simulink model "s_alqrd2"  (Simulink 4.00)
settings: Solver=ode45  SolverMode=SingleTasking  StartTime=0.0  StopTime=20  FixedStep=0.1  MaxStep=0.1  RelTol=1e-3  AbsTol=1e-6
values from neighbouring files (symbols this model uses):
  C = [Cp, zeros(1,ns)]    [akalm1.m]    (also in kalm1.m = my_sys1.c; kalm2.m = my_sys1.c; kalm3.m = my_sys1.c; kalm4.m = [eye(3,3), zeros(3,3)])
  F = K*(x_un/x_un(1))/kq1    [abeob1.m]    (also in akalm1.m = xp_un*alpha; alqr1.m = K*(x_un/x_un(1))/k1; alqrd1.m = K*(x_un/x_un(1))/k1; apol1.m = K*(x_un/x_un(1))/k1)
  k1 = K(1)    [alqr1.m]    (also in alqrd1.m; apol1.m; pol1.m = -2*a*T1-1-T1/T2; pol2.m = -2*a*T1-1-T1/T2)
  Ts = 0.5    [abeob1.m]    (also in akalm1.m = 0.25; alqrd1.m = 0.25; kalm2.m; kalm3.m)
settings Model: LastModifiedBy=Administrator  SaveTime=off  SaveOutput=off  LimitDataPoints=off  BlockReductionOpt=off

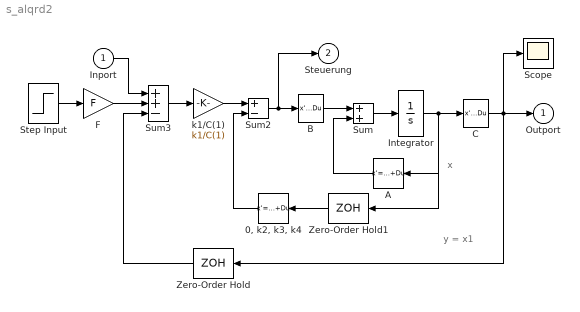
== system s_alqrd2 ==
  note: y = x1
  note: x
  Inport : Inport  Port=1
  "0, k2, k3, k4" : StateSpace  Orientation=left  A=[]  B=[]  C=[]  D=K  X0=0  Realization=auto  AbsoluteTolerance=auto  mask(Matrix Gain){@1=[0, k2, k3, k4]}
      mask prompts: @1 "Gain matrix:"
      mask help: Matrix Gain.
      mask init:
      | K = @1;
      mask Help: Multiplies input vector by entered matrix to produce output vector (y=Au).
      mask Display: disp('K')
  A : StateSpace  Orientation=left  A=[]  B=[]  C=[]  D=K  X0=0  Realization=auto  AbsoluteTolerance=auto  mask(Matrix Gain){@1=A}
      mask prompts: @1 "Gain matrix:"
      mask help: Matrix Gain.
      mask init:
      | K = @1;
      mask Help: Multiplies input vector by entered matrix to produce output vector (y=Au).
      mask Display: disp('K')
  B : StateSpace  A=[]  B=[]  C=[]  D=K  X0=0  Realization=auto  AbsoluteTolerance=auto  mask(Matrix Gain){@1=B}
      mask prompts: @1 "Gain matrix:"
      mask help: Matrix Gain.
      mask init:
      | K = @1;
      mask Help: Multiplies input vector by entered matrix to produce output vector (y=Au).
      mask Display: disp('K')
  C : StateSpace  A=[]  B=[]  C=[]  D=K  X0=0  Realization=auto  AbsoluteTolerance=auto  mask(Matrix Gain){@1=C}
      mask prompts: @1 "Gain matrix:"
      mask help: Matrix Gain.
      mask init:
      | K = @1;
      mask Help: Multiplies input vector by entered matrix to produce output vector (y=Au).
      mask Display: disp('K')
  F : Gain  Gain=F  Multiplication=Element-wise(K.*u)  SaturateOnIntegerOverflow=on
  Integrator : Integrator  ExternalReset=none  InitialConditionSource=internal  InitialCondition=[0 0 0 0]  LimitOutput=off  UpperSaturationLimit=inf  LowerSaturationLimit=-inf  ShowSaturationPort=off  ShowStatePort=off  AbsoluteTolerance=auto
  Scope : Scope
      settings: TickLabels=on  TimeRange=20.604000  YMin=-4.240000  YMax=4.240000  SaveToWorkspace=off  SaveName=ScopeData  DataFormat=Array  LimitDataPoints=on  MaxDataPoints=5000
  Step Input : Step  Time=2  Before=0  After=1  SampleTime=0
  Sum : Sum  Inputs=++  SaturateOnIntegerOverflow=on
  Sum2 : Sum  Inputs=+-  SaturateOnIntegerOverflow=on
  Sum3 : Sum  Inputs=++-  SaturateOnIntegerOverflow=on
  Zero-Order Hold : ZeroOrderHold  Orientation=left  SampleTime=Ts
  Zero-Order Hold1 : ZeroOrderHold  Orientation=left  SampleTime=Ts
  k1/C(1) : Gain  Gain=k1/C(1)  Multiplication=Element-wise(K.*u)  SaturateOnIntegerOverflow=on
  Outport : Outport  Port=1  InitialOutput=0
  Steuerung : Outport  Port=2  InitialOutput=0
  wires:
  Zero-Order Hold1/1 -> "0, k2, k3, k4"/1
  Zero-Order Hold/1 -> Sum3/3
  C/1 -> Scope/1, Zero-Order Hold/1, Outport/1
  Step Input/1 -> F/1
  F/1 -> Sum3/2
  Sum2/1 -> Steuerung/1, B/1
  Inport/1 -> Sum3/1
  Sum3/1 -> k1/C(1)/1
  k1/C(1)/1 -> Sum2/1
  "0, k2, k3, k4"/1 -> Sum2/2
  B/1 -> Sum/1
  A/1 -> Sum/2
  Sum/1 -> Integrator/1
  Integrator/1 -> Zero-Order Hold1/1, A/1, C/1
